simulink model "pm4_motor"  (R2017a)
settings: Solver=VariableStepAuto  StartTime=0.0  StopTime=3.0  RelTol=1e-3
libraries: simulink x1
settings Model: Creator=robotica  LastModifiedBy=robotica

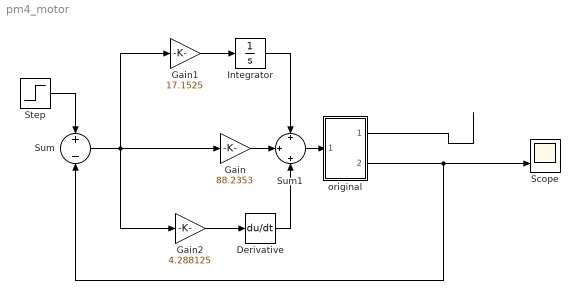
== system pm4_motor ==
  Derivative : Derivative
  Gain : Gain  Gain=88.2353
  Gain1 : Gain  Gain=17.1525
  Gain2 : Gain  Gain=4.288125
  Integrator : Integrator
  Scope : Scope  NumInputPorts=2
  Step : Step  SampleTime=1
  Sum : Sum  Inputs=+|-
  Sum1 : Sum  Inputs=+|+|+
  original : Subsystem
  wires:
  original/2(clean) -> Scope/2, Sum/2
  original/1(noisy) -> ?
  Sum/1 -> Gain2/1, Gain1/1, Gain/1
  Step/1 -> Sum/1
  Integrator/1 -> Sum1/1
  Gain/1 -> Sum1/2
  Sum1/1 -> original/1(signal)
  Gain1/1 -> Integrator/1
  Derivative/1 -> Sum1/3
  Gain2/1 -> Derivative/1

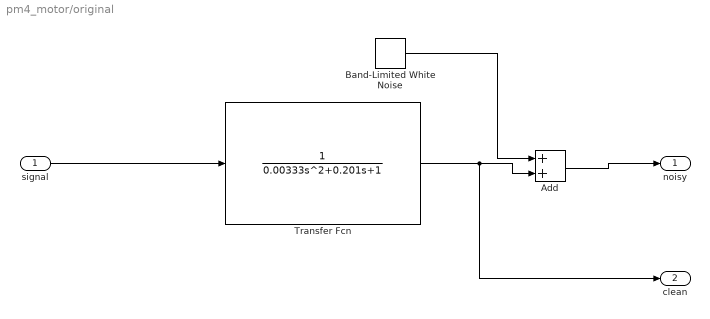
== system pm4_motor/original ==
  signal : Inport
  Add : Sum
  Band-Limited White Noise : simulink/Sources/Band-Limited White Noise  Cov=[0.0000001]  Ts=0.001  seed=[23341]
  Transfer Fcn : TransferFcn  Denominator=[0.00333 0.201 1]
  noisy : Outport
  clean : Outport  Port=2
  wires:
  Transfer Fcn/1 -> clean/1, Add/2
  Band-Limited White Noise/1 -> Add/1
  Add/1 -> noisy/1
  signal/1 -> Transfer Fcn/1
